simulink model "Openloop_"  (R2014a)
settings: Solver=ode45  StartTime=0.0  StopTime=50  RelTol=1e-3
settings Model: Creator=Hetram  LastModifiedBy=JATIN
settings DataIOCC: SignalLoggingSaveFormat=ModelDataLogs
settings OptimizationCC: ExpressionDepthLimit=2147483647
settings DebuggingCC: UnderspecifiedInitializationDetection=Classic  FcnCallInpInsideContextMsg=EnableAllAsWarning  StateNameClashWarn=warning

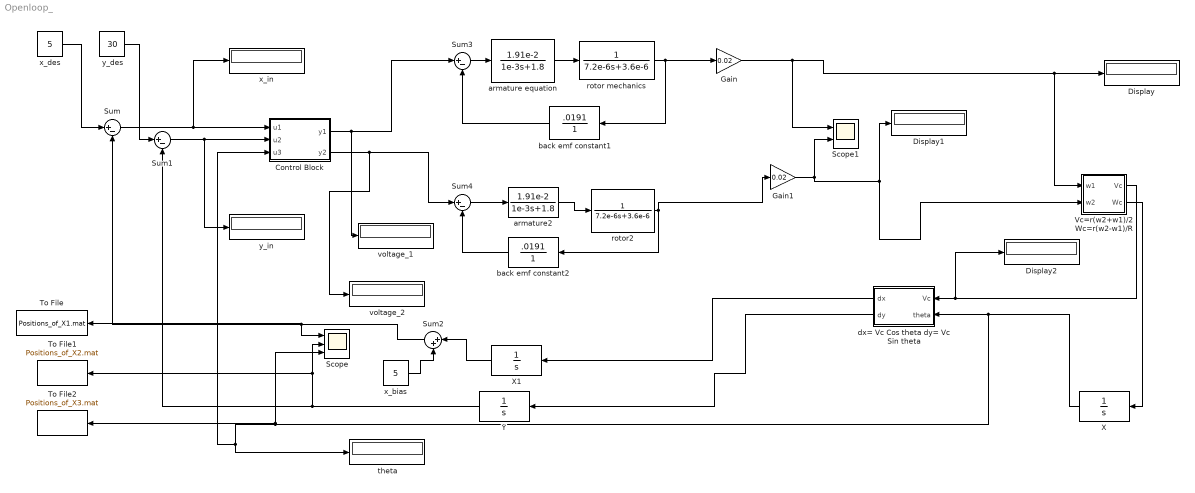
== system Openloop_ ==
  "Control Block " : MATLAB Function  TreatAsAtomicUnit=on
  Display : Display
  Display1 : Display
  Display2 : Display
  Gain : Gain  Gain=0.02
  Gain1 : Gain  Gain=0.02
  Scope : Scope  NumInputPorts=3
      settings: YMin=-5~-5~-5  YMax=5~5~5
  Scope1 : Scope  NumInputPorts=2
      settings: YMin=-5~-5  YMax=5~5
  Sum{,1,3..4} (4 alike) : Sum  Inputs=|+-
  Sum2 : Sum  Inputs=|++
  To File : ToFile  Filename=Positions_of_X1.mat  MatrixName=X_curr  SaveFormat=Timeseries
  To File1 : ToFile  Filename=Positions_of_X2.mat  MatrixName=Y_curr  SaveFormat=Timeseries
  To File2 : ToFile  Filename=Positions_of_X3.mat  MatrixName=theta  SaveFormat=Timeseries
  Vc=r(w2+w1)/2 Wc=r(w2-w1)/R : MATLAB Function  TreatAsAtomicUnit=on
  X : TransferFcn  Denominator=[1 0]
  X1 : TransferFcn  Denominator=[1 0]
  Y : TransferFcn  Denominator=[1 0]
  armature equation : TransferFcn  Numerator=[1.91e-2]  Denominator=[1e-3 1.8]
  armature2 : TransferFcn  Numerator=[1.91e-2]  Denominator=[1e-3 1.8]
  back emf constant1 : TransferFcn  Numerator=[.0191]  Denominator=[0 1]
  back emf constant2 : TransferFcn  Numerator=[.0191]  Denominator=[0 1]
  dx= Vc Cos theta dy= Vc Sin theta : MATLAB Function  TreatAsAtomicUnit=on
  rotor mechanics : TransferFcn  Denominator=[7.2e-6 3.6e-6]
  rotor2 : TransferFcn  Denominator=[7.2e-6 3.6e-6]
  theta : Display
  voltage_1 : Display
  voltage_2 : Display
  x_bias : Constant  Value=5
  x_des : Constant  Value=5
  x_in : Display
  y_des : Constant  Value=30
  y_in : Display
  wires:
  armature equation/1 -> rotor mechanics/1
  back emf constant1/1 -> Sum3/2
  Sum3/1 -> armature equation/1
  Sum4/1 -> armature2/1
  armature2/1 -> rotor2/1
  rotor2/1 -> Gain1/1, back emf constant2/1
  back emf constant2/1 -> Sum4/2
  "Control Block "/2(y2) -> voltage_2/1, Sum4/1
  Gain/1 -> Scope1/1, Display/1, Vc=r(w2+w1)/2 Wc=r(w2-w1)/R/1(w1)
  Gain1/1 -> Display1/1, Vc=r(w2+w1)/2 Wc=r(w2-w1)/R/2(w2), Scope1/2
  dx= Vc Cos theta dy= Vc Sin theta/2(dy) -> Y/1
  Vc=r(w2+w1)/2 Wc=r(w2-w1)/R/2(Wc) -> X/1
  rotor mechanics/1 -> back emf constant1/1, Gain/1
  Y/1 -> Sum1/2, To File1/1, Scope/2
  x_des/1 -> Sum/1
  y_des/1 -> Sum1/1
  Sum/1 -> x_in/1, "Control Block "/1(u1)
  Sum1/1 -> y_in/1, "Control Block "/2(u2)
  "Control Block "/1(y1) -> voltage_1/1, Sum3/1
  dx= Vc Cos theta dy= Vc Sin theta/1(dx) -> X1/1
  Vc=r(w2+w1)/2 Wc=r(w2-w1)/R/1(Vc) -> Display2/1, dx= Vc Cos theta dy= Vc Sin theta/1(Vc)
  x_bias/1 -> Sum2/2
  Sum2/1 -> Scope/1, To File/1, Sum/2
  X1/1 -> Sum2/1
  X/1 -> Scope/3, To File2/1, "Control Block "/3(u3), theta/1, dx= Vc Cos theta dy= Vc Sin theta/2(theta)

== matlab function Openloop_/dx= Vc Cos theta dy= Vc Sin theta ==
  data: Vc input; theta input; dx output; dy output
function [dx,dy] = fcn(Vc,theta)
%#codegen
dx=Vc*cos(theta);
dy=Vc*sin(theta);

== matlab function Openloop_/Vc=r(w2+w1)//2 Wc=r(w2-w1)//R ==
  data: w1 input; Vc output; w2 input; Wc output
function [Vc,Wc] = fcn(w1,w2)
%#codegen
r = 0.0508;
R = 0.24;
Vc = r*(w2+w1)/2;
Wc = r*(w2-w1)/R;

== matlab function Openloop_/Control Block  ==
  data: u1 input; y1 output; u2 input; u3 input; y2 output
function [y1,y2]= fcn(u1,u2,u3)
y1=0;
y2=0;
a=0;
%#codegen
x_des = 5;  
y_des = 30;

% x_des and y_des are to be fed in the refernce block as well
% Vw1 for Left wheel and Vw2 for Right Wheel
% Let voltages be of the limits 0-24 V positive as well as negative DC 

x_p = x_des - u1;
y_p = y_des - u2;
ang = u3 ;


if x_p==5 && y_p==0 && ang<(pi/2)
    y1 = -1;  
    y2 = 1; % Both the wheels are given forward motion        
elseif x_p>=0 && x_p<10 && y_p>=0 && y_p<35
    y1 = 2;  
    y2 = 2; % Both the wheels are given forward motion
elseif x_p>=0 && x_p<10 && y_p>=35 && y_p<45 && y1>=0 && y2>=0
    y1 = 24 - 2.4*(y_p-35);
    y2 = 24 - 2.4*(y_p-35);    % Speed Slow Down to zero

% elseif x_p>=0 && x_p<10 && y_p>=45 && y_p<50 && ang>=-1.57   
%     y1 =  12;
%     y2 = -12;    % Zero Turn towards right 
% 
% % elseif x_p>=0 && x_p<15 && y_p>=40 && y_p<50 && ang==-90 && y1<=24 && y2<=24
% %     y1 = 12 + 2.25*(x_p-5);
% %     y2 = 12 + 2.25*(x_p-5);    % Speed Increase to rated
% 
% elseif x_p>=10 && x_p<75 && y_p>=40 && y_p<50 && ang== -90 
%     y1 = 24;
%     y2 = 24;    % Both the wheels are given forward motion
% 
% elseif x_p>=75 && x_p<85 && y_p>=40 && y_p<50 && y1>=0 && y2>=0
%     y1 = 24 - 2.4*(x_p-50);
%     y2 = 24 - 2.4*(x_p-50);    % Speed Slow Down to zero
% 
% elseif x_p>=80 && x_p<90 && y_p>=40 && y_p<50 && ang<=90
%     y1 = -12;
%     y2 =  12;    % Zero Turn towards left    
% 
% % elseif x_p>=80 && x_p<90 && y_p>=40 && y_p<50 && ang==90 && y1<=24 && y2<=24
% %     y1 = 12 + 2.25*(x_p-25);
% %     y2 = 12 + 2.25*(x_p-25);    % Speed Increase to rated
% 
% elseif x_p>=80 && x_p<90 && y_p>=40 && y_p<100 && ang==0
%     y1 = 18;  
%     y2 = 18; % Both the wheels are given forward motion

end

    
     
% Angle aspect of motion is missing 
% Need to decide whether to put time delay for turns or angle feedback can
% be utilised 
end
